simulink model "Plant_2"  (R2024b)
settings: Solver=FixedStepAuto  StartTime=0.0  StopTime=20  FixedStep=0.02  RelTol=1e-3
values from neighbouring files (symbols this model uses):
  A = [ 0   1   0 ... (first row only)    [state_feedback_2.m]
  B = [ 0 ... (first row only)    [state_feedback_2.m]
  K = place(A, B, desired_poles)    [state_feedback_1.m]    (also in state_feedback_2.m = place(A,B,[p1 p2 p3]); state_feedback_3.m)
  K_r = -inv(E*inv(A-B*K)*B)    [state_feedback_3.m]
undefined symbols (not defined in the file or in its folder): L1, L2
settings Model: Creator=Sez26  LastModifiedBy=Sez26

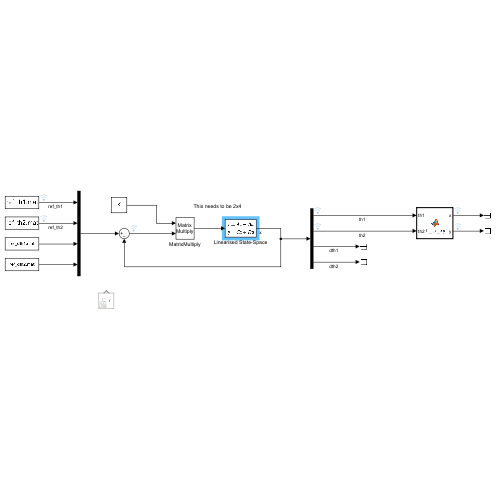
[thumbnail: Simulink's stored preview of the top-level diagram]
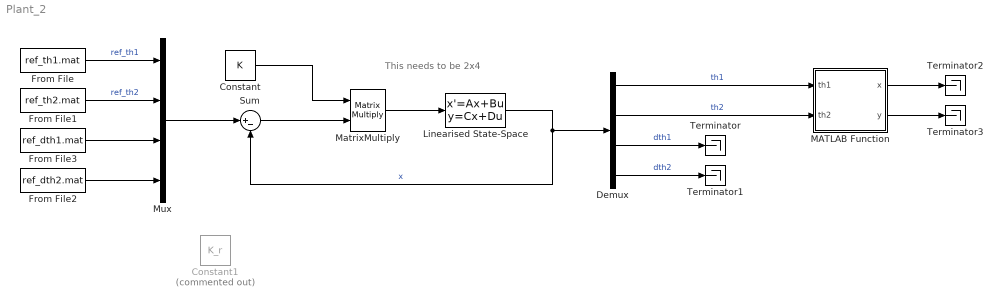
== system Plant_2 ==
  note: This needs to be 2x4
  Constant : Constant  Value=K
  Constant1 : Constant  Commented=on  Value=K_r
  Demux : Demux
  From File : FromFile  FileName=ref_th1.mat  SampleTime=0
  From File1 : FromFile  FileName=ref_th2.mat  SampleTime=0
  From File2 : FromFile  FileName=ref_dth2.mat  SampleTime=0
  From File3 : FromFile  FileName=ref_dth1.mat  SampleTime=0
  Linearised State-Space : StateSpace  A=A  B=B  C=[1 0 0 0; 0 1 0 0; 0 0 1 0; 0 0 0 1]  D=[0 0; 0 0; 0 0;0 0]  InitialCondition=0
  MATLAB Function : MATLAB Function  TreatAsAtomicUnit=on
  MatrixMultiply : Product  Multiplication=Matrix(*)
  Mux : Mux
  Sum : Sum  Inputs=|+-
  Terminator{,1..3} (4 alike) : Terminator
  wires:
  MATLAB Function/1(x) -> Terminator2/1
  MATLAB Function/2(y) -> Terminator3/1
  Linearised State-Space/1 -> Sum/2, Demux/1  "x"
  From File3/1 -> Mux/3
  From File2/1 -> Mux/4
  From File/1 -> Mux/1  "ref_th1"
  From File1/1 -> Mux/2  "ref_th2"
  Demux/3 -> Terminator/1  "dth1"
  Demux/4 -> Terminator1/1  "dth2"
  Demux/2 -> MATLAB Function/2(th2)  "th2"
  Demux/1 -> MATLAB Function/1(th1)  "th1"
  Mux/1 -> Sum/1
  Sum/1 -> MatrixMultiply/2
  MatrixMultiply/1 -> Linearised State-Space/1
  Constant/1 -> MatrixMultiply/1

== matlab function Plant_2/MATLAB Function ==
  data: x output; th1 input; y output; th2 input; L1 parameter; L2 parameter
function [x,y] = th_to_xy(th1, th2, L1, L2)
    x = L1*cos(deg2rad(th1)) + L2*cos(deg2rad(th2));
    y = L1*sin(deg2rad(th1)) + L2*sin(deg2rad(th2));
